simulink subsystem "API221_CustomMotion"  (R2022b)
settings: Solver=VariableStepAuto  StartTime=0.0  StopTime=10.0  RelTol=1e-3
settings Model: Creator=PROSTJP  LastModifiedBy=BEATOA

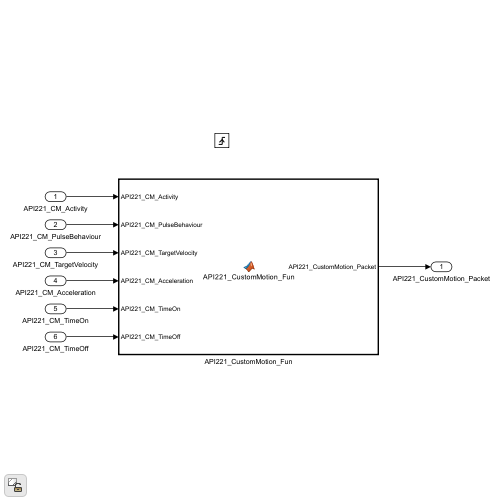
[thumbnail: Simulink's stored preview of the top-level diagram]
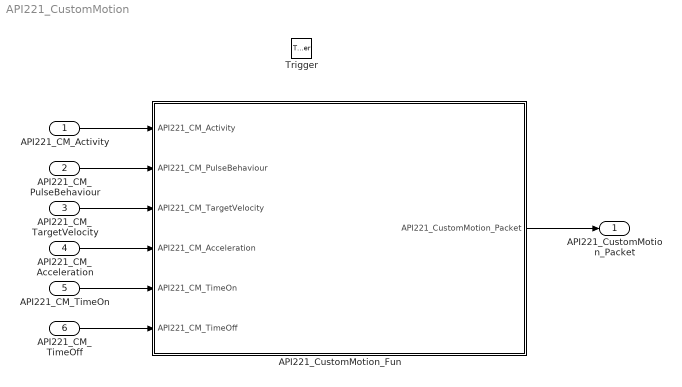
== system API221_CustomMotion ==
  API221_CM_Activity : Inport
  API221_CM_PulseBehaviour : Inport  Port=2
  API221_CM_TargetVelocity : Inport  Port=3
  API221_CM_Acceleration : Inport  Port=4
  API221_CM_TimeOn : Inport  Port=5
  API221_CM_TimeOff : Inport  Port=6
  Trigger : TriggerPort  VariantControl=(inherit)  PortDimensions=1
  API221_CustomMotion_Fun : MATLAB Function  TreatAsAtomicUnit=on
  API221_CustomMotion_Packet : Outport
  wires:
  API221_CustomMotion_Fun/1(API221_CustomMotion_Packet) -> API221_CustomMotion_Packet/1
  API221_CM_Acceleration/1 -> API221_CustomMotion_Fun/4(API221_CM_Acceleration)
  API221_CM_TimeOff/1 -> API221_CustomMotion_Fun/6(API221_CM_TimeOff)
  API221_CM_TargetVelocity/1 -> API221_CustomMotion_Fun/3(API221_CM_TargetVelocity)
  API221_CM_Activity/1 -> API221_CustomMotion_Fun/1(API221_CM_Activity)
  API221_CM_PulseBehaviour/1 -> API221_CustomMotion_Fun/2(API221_CM_PulseBehaviour)
  API221_CM_TimeOn/1 -> API221_CustomMotion_Fun/5(API221_CM_TimeOn)

== matlab function API221_CustomMotion/API221_CustomMotion_Fun ==
  data: API221_CustomMotion_Packet output uint8 [1..100]; API221_CM_Activity input; API221_CM_PulseBehaviour input; API221_CM_TargetVelocity input; API221_CM_Acceleration input; API221_CM_TimeOn input; API221_CM_TimeOff input
function API221_CustomMotion_Packet = API221_CustomMotion_Fun(API221_CM_Activity, API221_CM_PulseBehaviour, API221_CM_TargetVelocity, API221_CM_Acceleration, API221_CM_TimeOn, API221_CM_TimeOff)

     
    crc_dummy = 0; % Crc check on win packet not implemented
    PAD_SIZE = 100; 
    %sim_stop_time = 180;
    % API 221  - PULSE
    % HEADER
    destination = 0;
    node_id = 1;
    sdu_length = 11;
    sap = 4;
    api_id = 221;
    op_code = 6;
    cmd_fb = 0;
    frag = 0;
    mmp = 0;
    destination_source = destination + node_id * (2^4);
    opcode_compl = op_code + cmd_fb * (2^5) + frag * (2^6) + mmp * (2^7);

    motor_idx = uint8(0);
    
    header_api221 = uint8([destination_source sap sdu_length api_id opcode_compl]);
    
    API221_CustomMotion_Packet = zeros(PAD_SIZE,1,'uint8');


    switch (API221_CM_Activity)
        case 0
            % stop
            target_accel_arr = uint8([bitshift(API221_CM_Acceleration,-8), bitand(API221_CM_Acceleration,0x00FF)]);
            tmp = uint8([header_api221 motor_idx API221_CM_Activity target_accel_arr crc_dummy]);
            API221_CustomMotion_Packet(1:length(tmp)) = tmp(:);
        case 1
            % spin
            target_velocity_arr = uint8([bitshift(API221_CM_TargetVelocity,-8), bitand(API221_CM_TargetVelocity,0x00FF)]);
            target_accel_arr = uint8([bitshift(API221_CM_Acceleration,-8), bitand(API221_CM_Acceleration,0x00FF)]);
            tmp = uint8([header_api221 motor_idx API221_CM_Activity target_velocity_arr target_accel_arr crc_dummy]);
            API221_CustomMotion_Packet(1:length(tmp)) = tmp(:);
        case 2
            % pulse
            t_on_arr = uint8([bitand(API221_CM_TimeOn,0x00FF), bitshift(API221_CM_TimeOn,-8)]);
            t_off_arr = uint8([bitand(API221_CM_TimeOff,0x00FF), bitshift(API221_CM_TimeOff,-8)]);
            % check speed sign
            if API221_CM_TargetVelocity<0
                TargetVelocity = 256 + API221_CM_TargetVelocity;
            else
                TargetVelocity = API221_CM_TargetVelocity;
            end
            tmp = uint8([header_api221 motor_idx API221_CM_Activity API221_CM_PulseBehaviour TargetVelocity API221_CM_Acceleration t_on_arr t_off_arr crc_dummy]);
            API221_CustomMotion_Packet(1:length(tmp)) = tmp(:);
    end
